simulink model "Speed_Control"  (R2016a)
settings: Solver=VariableStepAuto  StartTime=0.0  StopTime=10.0  RelTol=1e-3
libraries: simulink x2
settings Model: Creator=USER  LastModifiedBy=dell
settings DebuggingCC: SFUnexpectedBacktrackingDiag=error  SFNoUnconditionalDefaultTransitionDiag=error
settings GRTTargetCC: TargetLangStandard=C99 (ISO)  GeneratePreprocessorConditionals=Use local settings
settings ConfigComp: CovMetricSettings=dwe  CovHtmlReporting=off  CovSaveCumulativeToWorkspaceVar=off  CovSaveSingleToWorkspaceVar=off  CovExternalEMLEnable=on

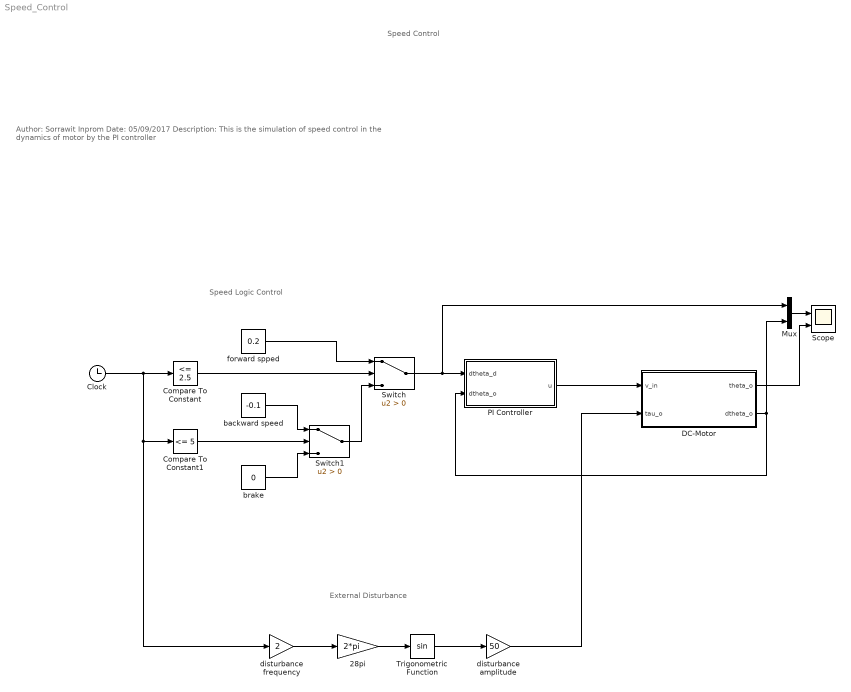
== system Speed_Control ==
  note: Speed Control
  note: Author: Sorrawit Inprom
      | Date: 05/09/2017
      | Description: This is the simulation of speed control in the dynamics of motor by the PI controller
  note: External Disturbance
  note: Speed Logic Control
  28pi : Gain  Gain=2*pi
  Clock : Clock
  Compare To Constant : simulink/Logic and Bit Operations/Compare To Constant  relop=<=  const=2.5  OutDataTypeStr=boolean
  Compare To Constant1 : simulink/Logic and Bit Operations/Compare To Constant  relop=<=  const=5  OutDataTypeStr=boolean
  DC-Motor : Subsystem
  Mux : Mux  Inputs=2
  PI Controller : Subsystem
  Scope : Scope  NumInputPorts=2
  Switch : Switch  Criteria=u2 > Threshold
  Switch1 : Switch  Criteria=u2 > Threshold
  Trigonometric Function : Trigonometry
  backward speed : Constant  Value=-0.1
  brake : Constant  Value=0
  disturbance amplitude : Gain  Gain=50
  disturbance frequency : Gain  Gain=2
  forward spped : Constant  Value=0.2
  wires:
  PI Controller/1(u) -> DC-Motor/1(v_in)
  Switch1/1 -> Switch/3
  forward spped/1 -> Switch/1
  backward speed/1 -> Switch1/1
  brake/1 -> Switch1/3
  Compare To Constant/1 -> Switch/2
  Compare To Constant1/1 -> Switch1/2
  Clock/1 -> Compare To Constant/1, Compare To Constant1/1, disturbance frequency/1
  disturbance frequency/1 -> 28pi/1
  28pi/1 -> Trigonometric Function/1
  Trigonometric Function/1 -> disturbance amplitude/1
  disturbance amplitude/1 -> DC-Motor/2(tau_o)
  Switch/1 -> Mux/1, PI Controller/1(dtheta_d)
  DC-Motor/2(dtheta_o) -> PI Controller/2(dtheta_o), Mux/2
  Mux/1 -> Scope/1
  DC-Motor/1(theta_o) -> Scope/2

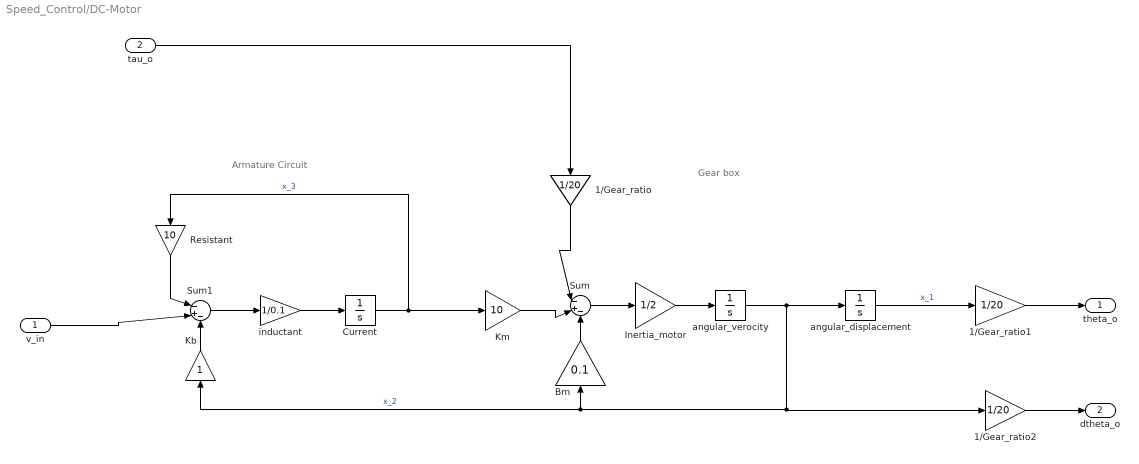
== system Speed_Control/DC-Motor ==
  note: Gear box
  note: Armature Circuit
  v_in : Inport
  tau_o : Inport  Port=2
  1/Gear_ratio : Gain  Gain=1/20
  1/Gear_ratio1 : Gain  Gain=1/20
  1/Gear_ratio2 : Gain  Gain=1/20
  "Bm " : Gain  Gain=0.1
  Current : Integrator
  Inertia_motor : Gain  Gain=1/2
  Kb : Gain
  Km : Gain  Gain=10
  "Resistant " : Gain  Gain=10
  Sum : Sum  Inputs=|-+-
  Sum1 : Sum  Inputs=|-+-
  angular_displacement : Integrator
  angular_verocity : Integrator
  inductant : Gain  Gain=1/0.1
  theta_o : Outport
  dtheta_o : Outport  Port=2
  wires:
  angular_displacement/1 -> 1/Gear_ratio1/1  "x_1"
  Current/1 -> Km/1, "Resistant "/1  "x_3"
  Inertia_motor/1 -> angular_verocity/1
  "Resistant "/1 -> Sum1/1
  1/Gear_ratio/1 -> Sum/1
  inductant/1 -> Current/1
  Sum1/1 -> inductant/1
  Sum/1 -> Inertia_motor/1
  Km/1 -> Sum/2
  "Bm "/1 -> Sum/3
  angular_verocity/1 -> "Bm "/1, Kb/1, 1/Gear_ratio2/1, angular_displacement/1  "x_2"
  Kb/1 -> Sum1/3
  v_in/1 -> Sum1/2
  tau_o/1 -> 1/Gear_ratio/1
  1/Gear_ratio1/1 -> theta_o/1
  1/Gear_ratio2/1 -> dtheta_o/1

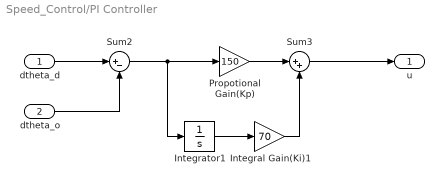
== system Speed_Control/PI Controller ==
  dtheta_d : Inport
  dtheta_o : Inport  Port=2
  Integral Gain(Ki)1 : Gain  Gain=70
  Integrator1 : Integrator
  Propotional Gain(Kp) : Gain  Gain=150
  Sum2 : Sum  Inputs=|+-
  Sum3 : Sum  Inputs=|++
  u : Outport
  wires:
  Integrator1/1 -> Integral Gain(Ki)1/1
  Propotional Gain(Kp)/1 -> Sum3/1
  Sum3/1 -> u/1
  dtheta_d/1 -> Sum2/1
  Integral Gain(Ki)1/1 -> Sum3/2
  dtheta_o/1 -> Sum2/2
  Sum2/1 -> Propotional Gain(Kp)/1, Integrator1/1
